simulink model "TestLevel_1_MODEL"  (R2017b)
settings: Solver=VariableStepAuto  StartTime=0.0  StopTime=30000000  RelTol=1e-3
libraries: instrumentlib x2, svdutilitieslib x1
settings Model: Creator=koch  LastModifiedBy=koch

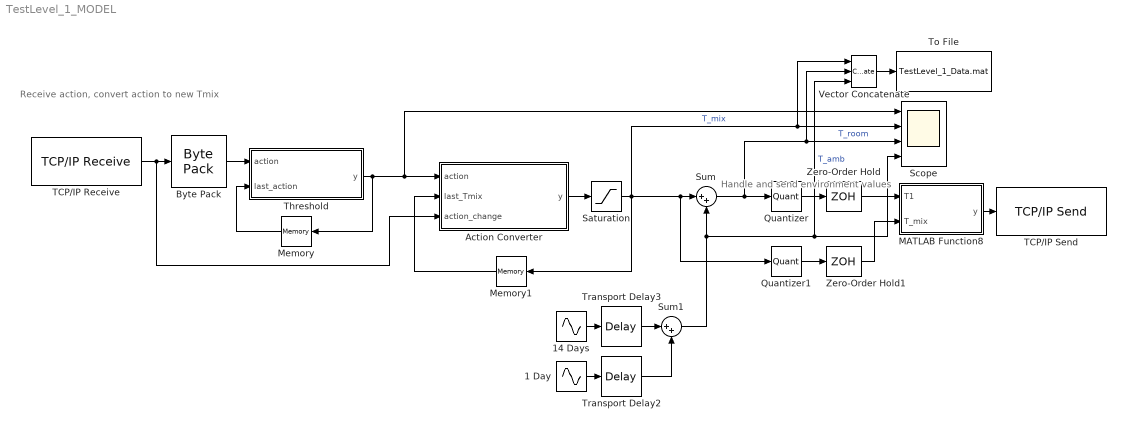
== system TestLevel_1_MODEL ==
  note: Receive action, convert action to new Tmix
  note: Handle and send environment values
  1 Day : Sin  Amplitude=4  Frequency=0.00007272205216643  SampleTime=0
  14 Days : Sin  Amplitude=2  Frequency=0.00000519443  SampleTime=0
  Action Converter : MATLAB Function  TreatAsAtomicUnit=on
  Byte Pack : svdutilitieslib/Byte Pack  datatypes={'uint8'}  byteAlign=1  blockPlatform=arduinoert
      settings: SourceProductName=Simulink Support Package for Arduino Hardware  SourceProductBaseCode=ARDUINO
  MATLAB Function8 : MATLAB Function  TreatAsAtomicUnit=on
  Memory : Memory
  Memory1 : Memory  InitialCondition=24
  Quantizer : Quantizer  QuantizationInterval=0.1
  Quantizer1 : Quantizer  QuantizationInterval=0.1
  Saturation : Saturate  UpperLimit=45  LowerLimit=15
  Scope : Scope  NumInputPorts=4
  Sum : Sum  Inputs=|++
  Sum1 : Sum  Inputs=|++
  TCP/IP Receive : instrumentlib/TCP//IP Receive  Host=localhost  Port=50000  DataSize=[1 1]  EnableBlockingMode=on  Timeout=20  SampleTime=200  DataType=uint8  ByteOrder=BigEndian
      settings: SourceProductName=Instrument Control Toolbox
  TCP/IP Send : instrumentlib/TCP//IP Send  Host=localhost  Port=50001  EnableBlockingMode=on  Timeout=10  ByteOrder=LittleEndian
      settings: SourceProductName=Instrument Control Toolbox
  Threshold : MATLAB Function  TreatAsAtomicUnit=on
  To File : ToFile  Filename=TestLevel_1_Data.mat  SaveFormat=Timeseries
  Transport Delay2 : TransportDelay  DelayTime=7000000
  Transport Delay3 : TransportDelay  DelayTime=5000000
  Vector Concatenate : Concatenate  NumInputs=3
  Zero-Order Hold : ZeroOrderHold  SampleTime=-1
  Zero-Order Hold1 : ZeroOrderHold  SampleTime=-1
  wires:
  Transport Delay3/1 -> Sum1/1
  Vector Concatenate/1 -> To File/1
  Memory/1 -> Threshold/2(last_action)
  MATLAB Function8/1(y) -> TCP/IP Send/1
  Quantizer/1 -> Zero-Order Hold/1
  Byte Pack/1 -> Threshold/1(action)
  Sum/1 -> Quantizer/1, Vector Concatenate/2, Scope/3  "T_room"
  Threshold/1(y) -> Action Converter/1(action), Scope/1, Memory/1
  Transport Delay2/1 -> Sum1/2
  Saturation/1 -> Quantizer1/1, Sum/1, Vector Concatenate/1, Scope/2, Memory1/1  "T_mix"
  TCP/IP Receive/1 -> Action Converter/3(action_change), Byte Pack/1
  Sum1/1 -> Scope/4, Vector Concatenate/3, Sum/2  "T_amb"
  Memory1/1 -> Action Converter/2(last_Tmix)
  Action Converter/1(y) -> Saturation/1
  Zero-Order Hold1/1 -> MATLAB Function8/2(T_mix)
  Quantizer1/1 -> Zero-Order Hold1/1
  Zero-Order Hold/1 -> MATLAB Function8/1(T1)
  14 Days/1 -> Transport Delay3/1
  1 Day/1 -> Transport Delay2/1

== matlab function TestLevel_1_MODEL/Action Converter ==
  data: action input; y output; last_Tmix input; action_change input
function y = fcn(action,last_Tmix,action_change)

if action_change > 0 
	k = 1;
else
    k = 0;
end


if action < 2 && k>0
    y = last_Tmix;
    k = 0;
elseif 1 < action && action < 3 && k>0
    y = last_Tmix -0.1;
    k = 0;
elseif 2 < action && k>0
    y = last_Tmix+0.5;
    k = 0;
elseif action > 20
    y = action;
else
    y=last_Tmix;
end

== matlab function TestLevel_1_MODEL/Threshold ==
  data: action input; y output; last_action input
function y  = fcn(action,last_action)

action = double(action);
% zero is not a option so
if action > 0
    y = action;
else
    y = last_action;
end

== matlab function TestLevel_1_MODEL/MATLAB Function8 ==
  data: T1 input; y output; T_mix input
function y = fcn(T1, T_mix)


y = [T1,4.5,4.6,4.7,T_mix,4.9];
